simulink model "LUT_kidney_30"  (R2023b)
settings: Solver=FixedStepAuto  StartTime=0  StopTime=10.1  FixedStep=Timegap  RelTol=1e-3
model workspace (MAT data in the model file):
  T1_input = 1.34
(part 3 of 3)

== system LUT_kidney_30/If Action Subsystem6/If Action Subsystem2/If Action Subsystem9/If Action Subsystem11 ==
  In1 : Inport
  Action Port : ActionPort  ActionPortLabel=elseif( u1 >= 1.905)
  LUT 1.91RR : Lookup_n-D  NumberOfTableDimensions=1  BreakpointsForDimension1=[413.2483;519.9897;610.675;704.3665;797.694;890.604;983.1818;1075.506;1167.638;1259.622;1351.49;1443.267;1534.971;1626.615;1718.21;1809.765;1901.286]  Table=[400;500;600;700;800;900;1000;1100;1200;1300;1400;1500;1600;1700;1800;1900;2000]  InternalRulePriority=Speed  RndMeth=Simplest
  Out1 : Outport
  wires:
  In1/1 -> LUT 1.91RR/1
  LUT 1.91RR/1 -> Out1/1

== system LUT_kidney_30/If Action Subsystem6/If Action Subsystem2/If Action Subsystem9/If Action Subsystem2 ==
  In1 : Inport
  Action Port : ActionPort  ActionPortLabel=else
  LUT 1.90RR : Lookup_n-D  NumberOfTableDimensions=1  BreakpointsForDimension1=[413.317;520.0649;610.7574;704.4636;797.8115;890.7462;983.3522;1075.708;1167.873;1259.891;1351.795;1443.609;1535.35;1627.033;1718.667;1810.261;1901.822]  Table=[400;500;600;700;800;900;1000;1100;1200;1300;1400;1500;1600;1700;1800;1900;2000]  InternalRulePriority=Speed  RndMeth=Simplest
  Out1 : Outport
  wires:
  In1/1 -> LUT 1.90RR/1
  LUT 1.90RR/1 -> Out1/1

== system LUT_kidney_30/If Action Subsystem6/If Action Subsystem2/If Action Subsystem9/If Action Subsystem3 ==
  In1 : Inport
  Action Port : ActionPort  ActionPortLabel=elseif( u1 >= 1.925)
  LUT 1.93RR : Lookup_n-D  NumberOfTableDimensions=1  BreakpointsForDimension1=[413.1126;519.8417;610.5139;704.1773;797.4656;890.3275;982.8502;1075.115;1167.182;1259.098;1350.896;1442.6;1534.23;1625.798;1717.317;1808.794;1900.237]  Table=[400;500;600;700;800;900;1000;1100;1200;1300;1400;1500;1600;1700;1800;1900;2000]  InternalRulePriority=Speed  RndMeth=Simplest
  Out1 : Outport
  wires:
  In1/1 -> LUT 1.93RR/1
  LUT 1.93RR/1 -> Out1/1

== system LUT_kidney_30/If Action Subsystem6/If Action Subsystem2/If Action Subsystem9/If Action Subsystem4 ==
  In1 : Inport
  Action Port : ActionPort  ActionPortLabel=elseif( u1 >= 1.935)
  LUT 1.94RR : Lookup_n-D  NumberOfTableDimensions=1  BreakpointsForDimension1=[413.0457;519.7691;610.4352;704.0852;797.3546;890.1931;982.6891;1074.924;1166.96;1258.843;1350.606;1442.275;1533.868;1625.4;1716.881;1808.32;1899.724]  Table=[400;500;600;700;800;900;1000;1100;1200;1300;1400;1500;1600;1700;1800;1900;2000]  InternalRulePriority=Speed  RndMeth=Simplest
  Out1 : Outport
  wires:
  In1/1 -> LUT 1.94RR/1
  LUT 1.94RR/1 -> Out1/1

== system LUT_kidney_30/If Action Subsystem6/If Action Subsystem2/If Action Subsystem9/If Action Subsystem5 ==
  In1 : Inport
  Action Port : ActionPort  ActionPortLabel=elseif( u1 >= 1.955)
  LUT 1.96RR : Lookup_n-D  NumberOfTableDimensions=1  BreakpointsForDimension1=[412.9134;519.6263;610.2812;703.9056;797.1386;889.9319;982.3757;1074.553;1166.527;1258.345;1350.041;1441.64;1533.162;1624.621;1716.028;1807.393;1898.722]  Table=[400;500;600;700;800;900;1000;1100;1200;1300;1400;1500;1600;1700;1800;1900;2000]  InternalRulePriority=Speed  RndMeth=Simplest
  Out1 : Outport
  wires:
  In1/1 -> LUT 1.96RR/1
  LUT 1.96RR/1 -> Out1/1

== system LUT_kidney_30/If Action Subsystem6/If Action Subsystem2/If Action Subsystem9/If Action Subsystem6 ==
  In1 : Inport
  Action Port : ActionPort  ActionPortLabel=elseif( u1 >= 1.945)
  LUT 1.95RR : Lookup_n-D  NumberOfTableDimensions=1  BreakpointsForDimension1=[412.9793;519.6973;610.3576;703.9946;797.2456;890.0613;982.5309;1074.737;1166.742;1258.592;1350.321;1441.955;1533.512;1625.007;1716.451;1807.853;1899.219]  Table=[400;500;600;700;800;900;1000;1100;1200;1300;1400;1500;1600;1700;1800;1900;2000]  InternalRulePriority=Speed  RndMeth=Simplest
  Out1 : Outport
  wires:
  In1/1 -> LUT 1.95RR/1
  LUT 1.95RR/1 -> Out1/1

== system LUT_kidney_30/If Action Subsystem6/If Action Subsystem2/If Action Subsystem9/If Action Subsystem7 ==
  In1 : Inport
  Action Port : ActionPort  ActionPortLabel=elseif( u1 >= 1.965)
  LUT 1.97RR : Lookup_n-D  NumberOfTableDimensions=1  BreakpointsForDimension1=[412.8481;519.5561;610.2059;703.8182;797.0336;889.8049;982.2233;1074.373;1166.317;1258.103;1349.766;1441.331;1532.818;1624.241;1715.612;1806.94;1898.232]  Table=[400;500;600;700;800;900;1000;1100;1200;1300;1400;1500;1600;1700;1800;1900;2000]  InternalRulePriority=Speed  RndMeth=Simplest
  Out1 : Outport
  wires:
  In1/1 -> LUT 1.97RR/1
  LUT 1.97RR/1 -> Out1/1

== system LUT_kidney_30/If Action Subsystem6/If Action Subsystem2/If Action Subsystem9/If Action Subsystem8 ==
  In1 : Inport
  Action Port : ActionPort  ActionPortLabel=elseif( u1 >= 1.975)
  LUT 1.98RR : Lookup_n-D  NumberOfTableDimensions=1  BreakpointsForDimension1=[412.7834;519.4867;610.1317;703.7323;796.9305;889.6803;982.0738;1074.196;1166.11;1257.865;1349.495;1441.026;1532.479;1623.867;1715.202;1806.494;1897.749]  Table=[400;500;600;700;800;900;1000;1100;1200;1300;1400;1500;1600;1700;1800;1900;2000]  InternalRulePriority=Speed  RndMeth=Simplest
  Out1 : Outport
  wires:
  In1/1 -> LUT 1.98RR/1
  LUT 1.98RR/1 -> Out1/1

== system LUT_kidney_30/If Action Subsystem6/If Action Subsystem2/If Action Subsystem9/If Action Subsystem9 ==
  In1 : Inport
  Action Port : ActionPort  ActionPortLabel=elseif(u1 >= 1.985)
  LUT 1.99RR : Lookup_n-D  NumberOfTableDimensions=1  BreakpointsForDimension1=[412.7191;519.4181;610.0586;703.6478;796.8293;889.5581;981.9271;1074.022;1165.907;1257.631;1349.229;1440.727;1532.145;1623.498;1714.798;1806.054;1897.273]  Table=[400;500;600;700;800;900;1000;1100;1200;1300;1400;1500;1600;1700;1800;1900;2000]  InternalRulePriority=Speed  RndMeth=Simplest
  Out1 : Outport
  wires:
  In1/1 -> LUT 1.99RR/1
  LUT 1.99RR/1 -> Out1/1

== system LUT_kidney_30/If Action Subsystem6/If Action Subsystem3/If Action Subsystem5/If Action Subsystem1 ==
  In1 : Inport
  Action Port : ActionPort  ActionPortLabel=elseif( u1 >= 0.615)
  LUT 0.62RR : Lookup_n-D  NumberOfTableDimensions=1  BreakpointsForDimension1=[428.1974;545.7526;646.9497;753.5478;860.9281;968.6199;1076.443;1184.289;1292.077;1399.741;1507.217;1614.398;1721.814;1828.354;1934.705;2040.709;2146.328]  Table=[400;500;600;700;800;900;1000;1100;1200;1300;1400;1500;1600;1700;1800;1900;2000]  InternalRulePriority=Speed  RndMeth=Simplest
  Out1 : Outport
  wires:
  In1/1 -> LUT 0.62RR/1
  LUT 0.62RR/1 -> Out1/1

== system LUT_kidney_30/If Action Subsystem6/If Action Subsystem3/If Action Subsystem5/If Action Subsystem10 ==
  In1 : Inport
  Action Port : ActionPort  ActionPortLabel=elseif( u1 >= 0.605)
  LUT 0.61RR : Lookup_n-D  NumberOfTableDimensions=1  BreakpointsForDimension1=[428.4312;545.8922;647.1097;753.8177;861.3559;969.2312;1077.248;1185.285;1293.251;1401.073;1508.677;1615.901;1723.325;1829.962;1936.285;2042.203;2147.679]  Table=[400;500;600;700;800;900;1000;1100;1200;1300;1400;1500;1600;1700;1800;1900;2000]  InternalRulePriority=Speed  RndMeth=Simplest
  Out1 : Outport
  wires:
  In1/1 -> LUT 0.61RR/1
  LUT 0.61RR/1 -> Out1/1

== system LUT_kidney_30/If Action Subsystem6/If Action Subsystem3/If Action Subsystem5/If Action Subsystem2 ==
  In1 : Inport
  Action Port : ActionPort  ActionPortLabel=else
  LUT 0.6RR : Lookup_n-D  NumberOfTableDimensions=1  BreakpointsForDimension1=[428.6987;546.0043;647.2017;753.9879;861.6572;969.6921;1077.879;1186.082;1294.201;1402.149;1509.845;1616.968;1724.511;1831.145;1937.377;2043.141;2148.399]  Table=[400;500;600;700;800;900;1000;1100;1200;1300;1400;1500;1600;1700;1800;1900;2000]  InternalRulePriority=Speed  RndMeth=Simplest
  Out1 : Outport
  wires:
  In1/1 -> LUT 0.6RR/1
  LUT 0.6RR/1 -> Out1/1

== system LUT_kidney_30/If Action Subsystem6/If Action Subsystem3/If Action Subsystem5/If Action Subsystem3 ==
  In1 : Inport
  Action Port : ActionPort  ActionPortLabel=elseif( u1 >= 0.625)
  LUT 0.63RR : Lookup_n-D  NumberOfTableDimensions=1  BreakpointsForDimension1=[427.9914;545.5872;646.7294;753.1904;860.3904;967.8787;1075.489;1183.124;1290.711;1398.191;1505.511;1612.588;1715.429;1826.388;1932.712;2038.744;2144.441]  Table=[400;500;600;700;800;900;1000;1100;1200;1300;1400;1500;1600;1700;1800;1900;2000]  InternalRulePriority=Speed  RndMeth=Simplest
  Out1 : Outport
  wires:
  In1/1 -> LUT 0.63RR/1
  LUT 0.63RR/1 -> Out1/1

== system LUT_kidney_30/If Action Subsystem6/If Action Subsystem3/If Action Subsystem5/If Action Subsystem4 ==
  In1 : Inport
  Action Port : ActionPort  ActionPortLabel=elseif( u1 >= 0.635)
  LUT 0.64RR : Lookup_n-D  NumberOfTableDimensions=1  BreakpointsForDimension1=[427.808;545.398;646.4556;752.7565;859.7576;967.026;1074.408;1181.814;1289.182;1396.459;1503.597;1610.531;1716.149;1824.126;1930.372;2036.381;2142.102]  Table=[400;500;600;700;800;900;1000;1100;1200;1300;1400;1500;1600;1700;1800;1900;2000]  InternalRulePriority=Speed  RndMeth=Simplest
  Out1 : Outport
  wires:
  In1/1 -> LUT 0.64RR/1
  LUT 0.64RR/1 -> Out1/1

== system LUT_kidney_30/If Action Subsystem6/If Action Subsystem3/If Action Subsystem5/If Action Subsystem5 ==
  In1 : Inport
  Action Port : ActionPort  ActionPortLabel=elseif( u1 >= 0.655)
  LUT 0.66RR : Lookup_n-D  NumberOfTableDimensions=1  BreakpointsForDimension1=[427.4919;544.956;645.7725;751.6992;858.2596;965.0507;1071.94;1178.854;1285.742;1392.564;1499.281;1605.85;1712.098;1818.958;1924.88;2030.721;2136.353]  Table=[400;500;600;700;800;900;1000;1100;1200;1300;1400;1500;1600;1700;1800;1900;2000]  InternalRulePriority=Speed  RndMeth=Simplest
  Out1 : Outport
  wires:
  In1/1 -> LUT 0.66RR/1
  LUT 0.66RR/1 -> Out1/1

== system LUT_kidney_30/If Action Subsystem6/If Action Subsystem3/If Action Subsystem5/If Action Subsystem6 ==
  In1 : Inport
  Action Port : ActionPort  ActionPortLabel=elseif( u1 >= 0.645)
  LUT 0.65RR : Lookup_n-D  NumberOfTableDimensions=1  BreakpointsForDimension1=[427.6427;545.187;646.1347;752.2564;859.0433;966.0784;1073.219;1180.384;1287.518;1394.574;1501.51;1608.272;1714.518;1821.628;1927.744;2033.688;2139.384]  Table=[400;500;600;700;800;900;1000;1100;1200;1300;1400;1500;1600;1700;1800;1900;2000]  InternalRulePriority=Speed  RndMeth=Simplest
  Out1 : Outport
  wires:
  In1/1 -> LUT 0.65RR/1
  LUT 0.65RR/1 -> Out1/1

== system LUT_kidney_30/If Action Subsystem6/If Action Subsystem3/If Action Subsystem5/If Action Subsystem7 ==
  In1 : Inport
  Action Port : ActionPort  ActionPortLabel=elseif( u1 >= 0.665)
  LUT 0.67RR : Lookup_n-D  NumberOfTableDimensions=1  BreakpointsForDimension1=[427.3522;544.7069;645.3744;751.0932;857.4171;963.9562;1070.586;1177.24;1283.874;1390.451;1496.937;1603.295;1709.417;1816.218;1921.825;2027.529;2133.063]  Table=[400;500;600;700;800;900;1000;1100;1200;1300;1400;1500;1600;1700;1800;1900;2000]  InternalRulePriority=Speed  RndMeth=Simplest
  Out1 : Outport
  wires:
  In1/1 -> LUT 0.67RR/1
  LUT 0.67RR/1 -> Out1/1

== system LUT_kidney_30/If Action Subsystem6/If Action Subsystem3/If Action Subsystem5/If Action Subsystem8 ==
  In1 : Inport
  Action Port : ActionPort  ActionPortLabel=elseif(u1 >= 0.675)
  LUT 0.68RR : Lookup_n-D  NumberOfTableDimensions=1  BreakpointsForDimension1=[427.2211;544.4415;644.9453;750.4458;856.5257;962.8065;1069.171;1175.56;1281.933;1388.256;1494.501;1600.635;1706.583;1808.339;1918.622;2024.158;2129.564]  Table=[400;500;600;700;800;900;1000;1100;1200;1300;1400;1500;1600;1700;1800;1900;2000]  InternalRulePriority=Speed  RndMeth=Simplest
  Out1 : Outport
  wires:
  In1/1 -> LUT 0.68RR/1
  LUT 0.68RR/1 -> Out1/1

== system LUT_kidney_30/If Action Subsystem6/If Action Subsystem3/If Action Subsystem5/If Action Subsystem9 ==
  In1 : Inport
  Action Port : ActionPort  ActionPortLabel=if(u1 >= 0.685)
  LUT 0.69RR : Lookup_n-D  NumberOfTableDimensions=1  BreakpointsForDimension1=[427.0963;544.1615;644.4895;749.7638;855.594;961.6121;1067.708;1173.828;1279.934;1385.997;1491.993;1597.893;1703.64;1808.121;1915.309;2020.646;2125.899]  Table=[400;500;600;700;800;900;1000;1100;1200;1300;1400;1500;1600;1700;1800;1900;2000]  InternalRulePriority=Speed  RndMeth=Simplest
  Out1 : Outport
  wires:
  In1/1 -> LUT 0.69RR/1
  LUT 0.69RR/1 -> Out1/1

== system LUT_kidney_30/If Action Subsystem6/If Action Subsystem3/If Action Subsystem6/If Action Subsystem1 ==
  In1 : Inport
  Action Port : ActionPort  ActionPortLabel=elseif( u1 >= 0.515)
  LUT 0.52RR : Lookup_n-D  NumberOfTableDimensions=1  BreakpointsForDimension1=[433.127;545.732;644.4138;749.8879;856.9387;964.7053;1072.719;1180.644;1288.21;1395.177;1501.479;1606.762;1710.998;1814.056;1915.832;2016.24;2115.209]  Table=[400;500;600;700;800;900;1000;1100;1200;1300;1400;1500;1600;1700;1800;1900;2000]  InternalRulePriority=Speed  RndMeth=Simplest
  Out1 : Outport
  wires:
  In1/1 -> LUT 0.52RR/1
  LUT 0.52RR/1 -> Out1/1

== system LUT_kidney_30/If Action Subsystem6/If Action Subsystem3/If Action Subsystem6/If Action Subsystem10 ==
  In1 : Inport
  Action Port : ActionPort  ActionPortLabel=elseif( u1 >= 0.505)
  LUT 0.51RR : Lookup_n-D  NumberOfTableDimensions=1  BreakpointsForDimension1=[434.1573;545.5433;643.469;748.408;855.0555;962.4819;1070.166;1177.73;1284.868;1391.294;1496.956;1601.467;1704.767;1806.718;1907.209;2006.145;2103.45]  Table=[400;500;600;700;800;900;1000;1100;1200;1300;1400;1500;1600;1700;1800;1900;2000]  InternalRulePriority=Speed  RndMeth=Simplest
  Out1 : Outport
  wires:
  In1/1 -> LUT 0.51RR/1
  LUT 0.51RR/1 -> Out1/1

== system LUT_kidney_30/If Action Subsystem6/If Action Subsystem3/If Action Subsystem6/If Action Subsystem2 ==
  In1 : Inport
  Action Port : ActionPort  ActionPortLabel=else
  LUT 0.50RR : Lookup_n-D  NumberOfTableDimensions=1  BreakpointsForDimension1=[435.351;545.3234;642.354;746.6394;852.778;959.7636;1067.016;1174.11;1280.701;1386.344;1491.327;1594.889;1697.058;1797.686;1896.653;1993.856;2089.217]  Table=[400;500;600;700;800;900;1000;1100;1200;1300;1400;1500;1600;1700;1800;1900;2000]  InternalRulePriority=Speed  RndMeth=Simplest
  Out1 : Outport
  wires:
  In1/1 -> LUT 0.50RR/1
  LUT 0.50RR/1 -> Out1/1

== system LUT_kidney_30/If Action Subsystem6/If Action Subsystem3/If Action Subsystem6/If Action Subsystem3 ==
  In1 : Inport
  Action Port : ActionPort  ActionPortLabel=elseif( u1 >= 0.525)
  LUT 0.53RR : Lookup_n-D  NumberOfTableDimensions=1  BreakpointsForDimension1=[432.2397;545.8873;645.2001;751.1029;858.4628;966.4802;1074.733;1182.923;1290.811;1398.189;1502.336;1610.911;1715.912;1819.885;1922.734;2024.382;2124.761]  Table=[400;500;600;700;800;900;1000;1100;1200;1300;1400;1500;1600;1700;1800;1900;2000]  InternalRulePriority=Speed  RndMeth=Simplest
  Out1 : Outport
  wires:
  In1/1 -> LUT 0.53RR/1
  LUT 0.53RR/1 -> Out1/1

== system LUT_kidney_30/If Action Subsystem6/If Action Subsystem3/If Action Subsystem6/If Action Subsystem4 ==
  In1 : Inport
  Action Port : ActionPort  ActionPortLabel=elseif( u1 >= 0.535)
  LUT 0.54RR : Lookup_n-D  NumberOfTableDimensions=1  BreakpointsForDimension1=[431.4769;546.0078;645.8393;752.0761;859.6613;967.8505;1076.263;1184.633;1292.75;1400.431;1506.235;1614.046;1719.658;1824.376;1928.112;2030.794;2132.358]  Table=[400;500;600;700;800;900;1000;1100;1200;1300;1400;1500;1600;1700;1800;1900;2000]  InternalRulePriority=Speed  RndMeth=Simplest
  Out1 : Outport
  wires:
  In1/1 -> LUT 0.54RR/1
  LUT 0.54RR/1 -> Out1/1

== system LUT_kidney_30/If Action Subsystem6/If Action Subsystem3/If Action Subsystem6/If Action Subsystem5 ==
  In1 : Inport
  Action Port : ActionPort  ActionPortLabel=elseif( u1 >= 0.555)
  LUT 0.56RR : Lookup_n-D  NumberOfTableDimensions=1  BreakpointsForDimension1=[430.26;546.1426;646.7222;753.384;861.2069;969.5394;1078.07;1186.589;1294.93;1402.952;1510.471;1617.742;1724.183;1829.965;1934.999;2039.223;2142.587]  Table=[400;500;600;700;800;900;1000;1100;1200;1300;1400;1500;1600;1700;1800;1900;2000]  InternalRulePriority=Speed  RndMeth=Simplest
  Out1 : Outport
  wires:
  In1/1 -> LUT 0.56RR/1
  LUT 0.56RR/1 -> Out1/1

== system LUT_kidney_30/If Action Subsystem6/If Action Subsystem3/If Action Subsystem6/If Action Subsystem6 ==
  In1 : Inport
  Action Port : ActionPort  ActionPortLabel=elseif( u1 >= 0.545)
  LUT 0.55RR : Lookup_n-D  NumberOfTableDimensions=1  BreakpointsForDimension1=[430.822;546.0929;646.343;752.8295;860.5661;968.8574;1077.36;1185.836;1294.1;1401.992;1509.171;1616.285;1722.373;1827.688;1932.145;2035.678;2138.23]  Table=[400;500;600;700;800;900;1000;1100;1200;1300;1400;1500;1600;1700;1800;1900;2000]  InternalRulePriority=Speed  RndMeth=Simplest
  Out1 : Outport
  wires:
  In1/1 -> LUT 0.55RR/1
  LUT 0.55RR/1 -> Out1/1

== system LUT_kidney_30/If Action Subsystem6/If Action Subsystem3/If Action Subsystem6/If Action Subsystem7 ==
  In1 : Inport
  Action Port : ActionPort  ActionPortLabel=elseif( u1 >= 0.565)
  LUT 0.57RR : Lookup_n-D  NumberOfTableDimensions=1  BreakpointsForDimension1=[429.7777;546.1575;646.9876;753.7593;861.6116;969.9322;1078.439;1186.944;1295.3;1403.385;1511.058;1618.528;1725.203;1831.337;1936.821;2041.598;2145.619]  Table=[400;500;600;700;800;900;1000;1100;1200;1300;1400;1500;1600;1700;1800;1900;2000]  InternalRulePriority=Speed  RndMeth=Simplest
  Out1 : Outport
  wires:
  In1/1 -> LUT 0.57RR/1
  LUT 0.57RR/1 -> Out1/1

== system LUT_kidney_30/If Action Subsystem6/If Action Subsystem3/If Action Subsystem6/If Action Subsystem8 ==
  In1 : Inport
  Action Port : ActionPort  ActionPortLabel=elseif(u1 >= 0.575)
  LUT 0.58RR : Lookup_n-D  NumberOfTableDimensions=1  BreakpointsForDimension1=[429.3634;546.1386;647.1496;753.9739;861.806;970.0689;1078.506;1186.949;1295.269;1403.356;1511.097;1614.73;1725.536;1831.922;1937.747;2042.953;2147.499]  Table=[400;500;600;700;800;900;1000;1100;1200;1300;1400;1500;1600;1700;1800;1900;2000]  InternalRulePriority=Speed  RndMeth=Simplest
  Out1 : Outport
  wires:
  In1/1 -> LUT 0.58RR/1
  LUT 0.58RR/1 -> Out1/1

== system LUT_kidney_30/If Action Subsystem6/If Action Subsystem3/If Action Subsystem6/If Action Subsystem9 ==
  In1 : Inport
  Action Port : ActionPort  ActionPortLabel=if(u1 >= 0.585)
  LUT 0.59RR : Lookup_n-D  NumberOfTableDimensions=1  BreakpointsForDimension1=[429.0068;546.087;647.218;754.0448;861.8139;969.9797;1078.308;1186.649;1294.887;1402.926;1510.67;1616.845;1725.276;1831.827;1937.896;2043.427;2148.379]  Table=[400;500;600;700;800;900;1000;1100;1200;1300;1400;1500;1600;1700;1800;1900;2000]  InternalRulePriority=Speed  RndMeth=Simplest
  Out1 : Outport
  wires:
  In1/1 -> LUT 0.59RR/1
  LUT 0.59RR/1 -> Out1/1

== system LUT_kidney_30/If Action Subsystem6/If Action Subsystem3/If Action Subsystem7/If Action Subsystem1 ==
  In1 : Inport
  Action Port : ActionPort  ActionPortLabel=elseif( u1 >= 0.715)
  LUT 0.72RR : Lookup_n-D  NumberOfTableDimensions=1  BreakpointsForDimension1=[426.7421;543.2502;643.001;747.566;852.6291;957.8477;1063.128;1168.429;1273.722;1378.988;1484.209;1589.366;1694.431;1799.282;1905.246;2009.576;2114.25]  Table=[400;500;600;700;800;900;1000;1100;1200;1300;1400;1500;1600;1700;1800;1900;2000]  InternalRulePriority=Speed  RndMeth=Simplest
  Out1 : Outport
  wires:
  In1/1 -> LUT 0.72RR/1
  LUT 0.72RR/1 -> Out1/1

== system LUT_kidney_30/If Action Subsystem6/If Action Subsystem3/If Action Subsystem7/If Action Subsystem10 ==
  In1 : Inport
  Action Port : ActionPort  ActionPortLabel=elseif( u1 >= 0.705)
  LUT 0.71RR : Lookup_n-D  NumberOfTableDimensions=1  BreakpointsForDimension1=[426.8582;543.5643;643.5139;748.3188;853.6393;959.1251;1064.678;1170.252;1275.817;1381.351;1486.833;1592.242;1697.543;1802.536;1908.533;2013.326;2118.212]  Table=[400;500;600;700;800;900;1000;1100;1200;1300;1400;1500;1600;1700;1800;1900;2000]  InternalRulePriority=Speed  RndMeth=Simplest
  Out1 : Outport
  wires:
  In1/1 -> LUT 0.71RR/1
  LUT 0.71RR/1 -> Out1/1

== system LUT_kidney_30/If Action Subsystem6/If Action Subsystem3/If Action Subsystem7/If Action Subsystem2 ==
  In1 : Inport
  Action Port : ActionPort  ActionPortLabel=else
  LUT 0.70RR : Lookup_n-D  NumberOfTableDimensions=1  BreakpointsForDimension1=[426.9758;543.8686;644.0112;749.053;854.6296;960.3823;1066.207;1172.055;1277.891;1383.691;1489.432;1595.089;1700.619;1805.628;1911.928;2017.025;2122.105]  Table=[400;500;600;700;800;900;1000;1100;1200;1300;1400;1500;1600;1700;1800;1900;2000]  InternalRulePriority=Speed  RndMeth=Simplest
  Out1 : Outport
  wires:
  In1/1 -> LUT 0.70RR/1
  LUT 0.70RR/1 -> Out1/1

== system LUT_kidney_30/If Action Subsystem6/If Action Subsystem3/If Action Subsystem7/If Action Subsystem3 ==
  In1 : Inport
  Action Port : ActionPort  ActionPortLabel=elseif( u1 >= 0.725)
  LUT 0.73RR : Lookup_n-D  NumberOfTableDimensions=1  BreakpointsForDimension1=[426.6267;542.9275;642.4753;746.7989;851.6044;956.5563;1061.566;1166.593;1271.616;1376.614;1481.572;1586.475;1691.298;1795.96;1896.303;2005.799;2110.242]  Table=[400;500;600;700;800;900;1000;1100;1200;1300;1400;1500;1600;1700;1800;1900;2000]  InternalRulePriority=Speed  RndMeth=Simplest
  Out1 : Outport
  wires:
  In1/1 -> LUT 0.73RR/1
  LUT 0.73RR/1 -> Out1/1

== system LUT_kidney_30/If Action Subsystem6/If Action Subsystem3/If Action Subsystem7/If Action Subsystem4 ==
  In1 : Inport
  Action Port : ActionPort  ActionPortLabel=elseif( u1 >= 0.735)
  LUT 0.74RR : Lookup_n-D  NumberOfTableDimensions=1  BreakpointsForDimension1=[426.5109;542.5976;641.9396;746.0211;850.5697;955.2565;1059.996;1164.753;1269.505;1374.236;1478.933;1583.58;1688.158;1792.608;1895.708;2002.02;2106.209]  Table=[400;500;600;700;800;900;1000;1100;1200;1300;1400;1500;1600;1700;1800;1900;2000]  InternalRulePriority=Speed  RndMeth=Simplest
  Out1 : Outport
  wires:
  In1/1 -> LUT 0.74RR/1
  LUT 0.74RR/1 -> Out1/1

== system LUT_kidney_30/If Action Subsystem6/If Action Subsystem3/If Action Subsystem7/If Action Subsystem5 ==
  In1 : Inport
  Action Port : ActionPort  ActionPortLabel=elseif( u1 >= 0.755)
  LUT 0.76RR : Lookup_n-D  NumberOfTableDimensions=1  BreakpointsForDimension1=[426.2764;541.9209;640.8473;744.4465;848.4866;952.6498;1056.858;1161.081;1265.3;1369.502;1473.677;1577.814;1681.897;1785.894;1889.567;1994.603;2098.14]  Table=[400;500;600;700;800;900;1000;1100;1200;1300;1400;1500;1600;1700;1800;1900;2000]  InternalRulePriority=Speed  RndMeth=Simplest
  Out1 : Outport
  wires:
  In1/1 -> LUT 0.76RR/1
  LUT 0.76RR/1 -> Out1/1

== system LUT_kidney_30/If Action Subsystem6/If Action Subsystem3/If Action Subsystem7/If Action Subsystem6 ==
  In1 : Inport
  Action Port : ActionPort  ActionPortLabel=elseif( u1 >= 0.745)
  LUT 0.75RR : Lookup_n-D  NumberOfTableDimensions=1  BreakpointsForDimension1=[426.3943;542.2617;641.3963;745.236;849.5293;953.9529;1058.426;1162.914;1267.398;1371.864;1476.298;1580.69;1685.021;1789.248;1892.908;1998.271;2102.17]  Table=[400;500;600;700;800;900;1000;1100;1200;1300;1400;1500;1600;1700;1800;1900;2000]  InternalRulePriority=Speed  RndMeth=Simplest
  Out1 : Outport
  wires:
  In1/1 -> LUT 0.75RR/1
  LUT 0.75RR/1 -> Out1/1

== system LUT_kidney_30/If Action Subsystem6/If Action Subsystem3/If Action Subsystem7/If Action Subsystem7 ==
  In1 : Inport
  Action Port : ActionPort  ActionPortLabel=elseif( u1 >= 0.765)
  LUT 0.77RR : Lookup_n-D  NumberOfTableDimensions=1  BreakpointsForDimension1=[426.1567;541.5762;640.2948;743.6552;847.4448;951.3508;1055.298;1159.259;1263.215;1367.157;1471.074;1574.958;1678.795;1782.558;1886.105;1991.154;2094.134]  Table=[400;500;600;700;800;900;1000;1100;1200;1300;1400;1500;1600;1700;1800;1900;2000]  InternalRulePriority=Speed  RndMeth=Simplest
  Out1 : Outport
  wires:
  In1/1 -> LUT 0.77RR/1
  LUT 0.77RR/1 -> Out1/1

== system LUT_kidney_30/If Action Subsystem6/If Action Subsystem3/If Action Subsystem7/If Action Subsystem8 ==
  In1 : Inport
  Action Port : ActionPort  ActionPortLabel=elseif(u1 >= 0.775)
  LUT 0.78RR : Lookup_n-D  NumberOfTableDimensions=1  BreakpointsForDimension1=[426.035;541.2285;639.7402;742.8643;846.4065;950.0589;1053.749;1157.451;1261.149;1364.833;1468.496;1572.128;1675.719;1779.247;1882.619;1988.504;2090.168]  Table=[400;500;600;700;800;900;1000;1100;1200;1300;1400;1500;1600;1700;1800;1900;2000]  InternalRulePriority=Speed  RndMeth=Simplest
  Out1 : Outport
  wires:
  In1/1 -> LUT 0.78RR/1
  LUT 0.78RR/1 -> Out1/1

== system LUT_kidney_30/If Action Subsystem6/If Action Subsystem3/If Action Subsystem7/If Action Subsystem9 ==
  In1 : Inport
  Action Port : ActionPort  ActionPortLabel=if(u1 >= 0.785)
  LUT 0.79RR : Lookup_n-D  NumberOfTableDimensions=1  BreakpointsForDimension1=[425.9113;540.8787;639.1852;742.0757;845.3741;948.7768;1052.214;1155.661;1259.104;1362.535;1465.946;1569.329;1672.676;1775.969;1879.142;1980.779;2086.259]  Table=[400;500;600;700;800;900;1000;1100;1200;1300;1400;1500;1600;1700;1800;1900;2000]  InternalRulePriority=Speed  RndMeth=Simplest
  Out1 : Outport
  wires:
  In1/1 -> LUT 0.79RR/1
  LUT 0.79RR/1 -> Out1/1

== system LUT_kidney_30/If Action Subsystem6/If Action Subsystem3/If Action Subsystem8/If Action Subsystem1 ==
  In1 : Inport
  Action Port : ActionPort  ActionPortLabel=elseif( u1 >= 0.815)
  LUT 0.82RR : Lookup_n-D  NumberOfTableDimensions=1  BreakpointsForDimension1=[425.5456;539.8244;637.5294;739.7402;842.3309;945.0098;1047.714;1150.423;1253.127;1355.82;1458.498;1561.156;1663.787;1766.382;1868.911;1971.209;2075.321]  Table=[400;500;600;700;800;900;1000;1100;1200;1300;1400;1500;1600;1700;1800;1900;2000]  InternalRulePriority=Speed  RndMeth=Simplest
  Out1 : Outport
  wires:
  In1/1 -> LUT 0.82RR/1
  LUT 0.82RR/1 -> Out1/1

== system LUT_kidney_30/If Action Subsystem6/If Action Subsystem3/If Action Subsystem8/If Action Subsystem10 ==
  In1 : Inport
  Action Port : ActionPort  ActionPortLabel=elseif( u1 >= 0.805)
  LUT 0.81RR : Lookup_n-D  NumberOfTableDimensions=1  BreakpointsForDimension1=[425.6571;540.176;638.0787;740.5124;843.3348;946.2505;1049.195;1152.145;1255.091;1358.026;1460.944;1563.84;1666.707;1769.532;1872.279;1974.668;2078.739]  Table=[400;500;600;700;800;900;1000;1100;1200;1300;1400;1500;1600;1700;1800;1900;2000]  InternalRulePriority=Speed  RndMeth=Simplest
  Out1 : Outport
  wires:
  In1/1 -> LUT 0.81RR/1
  LUT 0.81RR/1 -> Out1/1

== system LUT_kidney_30/If Action Subsystem6/If Action Subsystem3/If Action Subsystem8/If Action Subsystem2 ==
  In1 : Inport
  Action Port : ActionPort  ActionPortLabel=else
  LUT 0.80RR : Lookup_n-D  NumberOfTableDimensions=1  BreakpointsForDimension1=[425.7853;540.5277;638.6309;741.2913;844.3496;947.5067;1050.695;1153.892;1257.084;1360.265;1463.427;1566.566;1669.671;1772.729;1875.692;1978.009;2082.433]  Table=[400;500;600;700;800;900;1000;1100;1200;1300;1400;1500;1600;1700;1800;1900;2000]  InternalRulePriority=Speed  RndMeth=Simplest
  Out1 : Outport
  wires:
  In1/1 -> LUT 0.80RR/1
  LUT 0.80RR/1 -> Out1/1

== system LUT_kidney_30/If Action Subsystem6/If Action Subsystem3/If Action Subsystem8/If Action Subsystem3 ==
  In1 : Inport
  Action Port : ActionPort  ActionPortLabel=elseif( u1 >= 0.825)
  LUT 0.83RR : Lookup_n-D  NumberOfTableDimensions=1  BreakpointsForDimension1=[425.3766;539.4735;636.984;738.976;841.3394;943.7861;1046.255;1148.727;1251.194;1353.65;1456.092;1558.515;1660.914;1763.28;1865.591;1967.739;2072.782]  Table=[400;500;600;700;800;900;1000;1100;1200;1300;1400;1500;1600;1700;1800;1900;2000]  InternalRulePriority=Speed  RndMeth=Simplest
  Out1 : Outport
  wires:
  In1/1 -> LUT 0.83RR/1
  LUT 0.83RR/1 -> Out1/1

== system LUT_kidney_30/If Action Subsystem6/If Action Subsystem3/If Action Subsystem8/If Action Subsystem4 ==
  In1 : Inport
  Action Port : ActionPort  ActionPortLabel=elseif( u1 >= 0.835)
  LUT 0.84RR : Lookup_n-D  NumberOfTableDimensions=1  BreakpointsForDimension1=[425.2593;539.1237;636.4432;738.2206;840.3612;942.5802;1044.819;1147.059;1249.293;1351.516;1453.726;1555.918;1658.089;1760.23;1862.324;1964.296;2064.45]  Table=[400;500;600;700;800;900;1000;1100;1200;1300;1400;1500;1600;1700;1800;1900;2000]  InternalRulePriority=Speed  RndMeth=Simplest
  Out1 : Outport
  wires:
  In1/1 -> LUT 0.84RR/1
  LUT 0.84RR/1 -> Out1/1

== system LUT_kidney_30/If Action Subsystem6/If Action Subsystem3/If Action Subsystem8/If Action Subsystem5 ==
  In1 : Inport
  Action Port : ActionPort  ActionPortLabel=elseif( u1 >= 0.855)
  LUT 0.86RR : Lookup_n-D  NumberOfTableDimensions=1  BreakpointsForDimension1=[424.9841;538.4295;635.3782;736.7393;838.4479;940.2258;1042.018;1143.808;1245.59;1347.362;1449.12;1550.864;1652.589;1754.29;1855.955;1957.544;2058.724]  Table=[400;500;600;700;800;900;1000;1100;1200;1300;1400;1500;1600;1700;1800;1900;2000]  InternalRulePriority=Speed  RndMeth=Simplest
  Out1 : Outport
  wires:
  In1/1 -> LUT 0.86RR/1
  LUT 0.86RR/1 -> Out1/1

== system LUT_kidney_30/If Action Subsystem6/If Action Subsystem3/If Action Subsystem8/If Action Subsystem6 ==
  In1 : Inport
  Action Port : ActionPort  ActionPortLabel=elseif( u1 >= 0.845)
  LUT 0.85RR : Lookup_n-D  NumberOfTableDimensions=1  BreakpointsForDimension1=[425.1226;538.7756;635.9078;737.4748;839.3971;941.3933;1043.406;1145.419;1247.424;1349.42;1451.402;1553.368;1655.313;1757.233;1859.111;1960.895;2061.924]  Table=[400;500;600;700;800;900;1000;1100;1200;1300;1400;1500;1600;1700;1800;1900;2000]  InternalRulePriority=Speed  RndMeth=Simplest
  Out1 : Outport
  wires:
  In1/1 -> LUT 0.85RR/1
  LUT 0.85RR/1 -> Out1/1

== system LUT_kidney_30/If Action Subsystem6/If Action Subsystem3/If Action Subsystem8/If Action Subsystem7 ==
  In1 : Inport
  Action Port : ActionPort  ActionPortLabel=elseif( u1 >= 0.865)
  LUT 0.87RR : Lookup_n-D  NumberOfTableDimensions=1  BreakpointsForDimension1=[424.8438;538.0859;634.8549;736.0145;837.5141;939.0785;1040.654;1142.226;1243.789;1345.342;1446.882;1548.407;1649.915;1751.402;1852.856;1954.248;2055.383]  Table=[400;500;600;700;800;900;1000;1100;1200;1300;1400;1500;1600;1700;1800;1900;2000]  InternalRulePriority=Speed  RndMeth=Simplest
  Out1 : Outport
  wires:
  In1/1 -> LUT 0.87RR/1
  LUT 0.87RR/1 -> Out1/1

== system LUT_kidney_30/If Action Subsystem6/If Action Subsystem3/If Action Subsystem8/If Action Subsystem8 ==
  In1 : Inport
  Action Port : ActionPort  ActionPortLabel=elseif(u1 >= 0.875)
  LUT 0.88RR : Lookup_n-D  NumberOfTableDimensions=1  BreakpointsForDimension1=[424.7021;537.7451;634.3384;735.301;836.596;937.9516;1039.316;1140.674;1242.024;1343.362;1444.687;1545.999;1647.294;1748.569;1849.816;1951.011;2052.028]  Table=[400;500;600;700;800;900;1000;1100;1200;1300;1400;1500;1600;1700;1800;1900;2000]  InternalRulePriority=Speed  RndMeth=Simplest
  Out1 : Outport
  wires:
  In1/1 -> LUT 0.88RR/1
  LUT 0.88RR/1 -> Out1/1

== system LUT_kidney_30/If Action Subsystem6/If Action Subsystem3/If Action Subsystem8/If Action Subsystem9 ==
  In1 : Inport
  Action Port : ActionPort  ActionPortLabel=if(u1 >= 0.885)
  LUT 0.89RR : Lookup_n-D  NumberOfTableDimensions=1  BreakpointsForDimension1=[424.5589;537.4073;633.829;734.5989;835.6941;936.8455;1038.003;1139.153;1240.292;1341.42;1442.536;1543.638;1644.724;1745.792;1846.835;1947.833;2048.701]  Table=[400;500;600;700;800;900;1000;1100;1200;1300;1400;1500;1600;1700;1800;1900;2000]  InternalRulePriority=Speed  RndMeth=Simplest
  Out1 : Outport
  wires:
  In1/1 -> LUT 0.89RR/1
  LUT 0.89RR/1 -> Out1/1

== system LUT_kidney_30/If Action Subsystem6/If Action Subsystem3/If Action Subsystem9/If Action Subsystem1 ==
  In1 : Inport
  Action Port : ActionPort  ActionPortLabel=elseif( u1 >= 0.915)
  LUT 0.92RR : Lookup_n-D  NumberOfTableDimensions=1  BreakpointsForDimension1=[424.1226;536.4147;632.346;732.5645;833.0871;933.6531;1034.217;1134.768;1235.305;1335.83;1436.341;1536.839;1637.324;1737.794;1838.244;1938.664;2039.021]  Table=[400;500;600;700;800;900;1000;1100;1200;1300;1400;1500;1600;1700;1800;1900;2000]  InternalRulePriority=Speed  RndMeth=Simplest
  Out1 : Outport
  wires:
  In1/1 -> LUT 0.92RR/1
  LUT 0.92RR/1 -> Out1/1

== system LUT_kidney_30/If Action Subsystem6/If Action Subsystem3/If Action Subsystem9/If Action Subsystem10 ==
  In1 : Inport
  Action Port : ActionPort  ActionPortLabel=elseif( u1 >= 0.905)
  LUT 0.91RR : Lookup_n-D  NumberOfTableDimensions=1  BreakpointsForDimension1=[424.269;536.7419;632.8326;733.2306;833.9395;934.6962;1035.453;1136.199;1236.933;1337.654;1438.363;1539.058;1639.74;1740.405;1841.049;1941.659;2042.191]  Table=[400;500;600;700;800;900;1000;1100;1200;1300;1400;1500;1600;1700;1800;1900;2000]  InternalRulePriority=Speed  RndMeth=Simplest
  Out1 : Outport
  wires:
  In1/1 -> LUT 0.91RR/1
  LUT 0.91RR/1 -> Out1/1

== system LUT_kidney_30/If Action Subsystem6/If Action Subsystem3/If Action Subsystem9/If Action Subsystem2 ==
  In1 : Inport
  Action Port : ActionPort  ActionPortLabel=else
  LUT 0.90RR : Lookup_n-D  NumberOfTableDimensions=1  BreakpointsForDimension1=[424.4145;537.0728;633.327;733.9087;834.8086;935.7603;1036.715;1137.661;1238.596;1339.518;1440.428;1541.324;1642.206;1743.071;1843.912;1944.716;2045.419]  Table=[400;500;600;700;800;900;1000;1100;1200;1300;1400;1500;1600;1700;1800;1900;2000]  InternalRulePriority=Speed  RndMeth=Simplest
  Out1 : Outport
  wires:
  In1/1 -> LUT 0.90RR/1
  LUT 0.90RR/1 -> Out1/1

== system LUT_kidney_30/If Action Subsystem6/If Action Subsystem3/If Action Subsystem9/If Action Subsystem3 ==
  In1 : Inport
  Action Port : ActionPort  ActionPortLabel=elseif( u1 >= 0.925)
  LUT 0.93RR : Lookup_n-D  NumberOfTableDimensions=1  BreakpointsForDimension1=[423.9754;536.0914;631.8672;731.9107;832.2512;932.6309;1033.005;1133.366;1233.712;1334.043;1434.361;1534.667;1634.959;1735.237;1835.496;1935.73;2035.91]  Table=[400;500;600;700;800;900;1000;1100;1200;1300;1400;1500;1600;1700;1800;1900;2000]  InternalRulePriority=Speed  RndMeth=Simplest
  Out1 : Outport
  wires:
  In1/1 -> LUT 0.93RR/1
  LUT 0.93RR/1 -> Out1/1

== system LUT_kidney_30/If Action Subsystem6/If Action Subsystem3/If Action Subsystem9/If Action Subsystem4 ==
  In1 : Inport
  Action Port : ActionPort  ActionPortLabel=elseif( u1 >= 0.935)
  LUT 0.94RR : Lookup_n-D  NumberOfTableDimensions=1  BreakpointsForDimension1=[423.8275;535.7721;631.3965;731.2692;831.4319;931.6296;1031.819;1131.993;1232.151;1332.294;1432.424;1532.54;1632.644;1732.734;1832.806;1932.855;2032.86]  Table=[400;500;600;700;800;900;1000;1100;1200;1300;1400;1500;1600;1700;1800;1900;2000]  InternalRulePriority=Speed  RndMeth=Simplest
  Out1 : Outport
  wires:
  In1/1 -> LUT 0.94RR/1
  LUT 0.94RR/1 -> Out1/1

== system LUT_kidney_30/If Action Subsystem6/If Action Subsystem3/If Action Subsystem9/If Action Subsystem5 ==
  In1 : Inport
  Action Port : ActionPort  ActionPortLabel=elseif( u1 >= 0.955)
  LUT 0.96RR : Lookup_n-D  NumberOfTableDimensions=1  BreakpointsForDimension1=[423.5306;535.146;630.4794;730.0228;829.8425;929.6888;1029.522;1129.335;1229.13;1328.908;1428.672;1528.423;1628.16;1727.885;1827.595;1927.285;2026.942]  Table=[400;500;600;700;800;900;1000;1100;1200;1300;1400;1500;1600;1700;1800;1900;2000]  InternalRulePriority=Speed  RndMeth=Simplest
  Out1 : Outport
  wires:
  In1/1 -> LUT 0.96RR/1
  LUT 0.96RR/1 -> Out1/1

== system LUT_kidney_30/If Action Subsystem6/If Action Subsystem3/If Action Subsystem9/If Action Subsystem6 ==
  In1 : Inport
  Action Port : ActionPort  ActionPortLabel=elseif( u1 >= 0.945)
  LUT 0.95RR : Lookup_n-D  NumberOfTableDimensions=1  BreakpointsForDimension1=[423.6792;535.4569;630.9339;730.6399;830.629;930.649;1030.658;1130.65;1230.624;1330.583;1430.528;1530.459;1630.378;1730.283;1830.173;1930.041;2029.871]  Table=[400;500;600;700;800;900;1000;1100;1200;1300;1400;1500;1600;1700;1800;1900;2000]  InternalRulePriority=Speed  RndMeth=Simplest
  Out1 : Outport
  wires:
  In1/1 -> LUT 0.95RR/1
  LUT 0.95RR/1 -> Out1/1

== system LUT_kidney_30/If Action Subsystem6/If Action Subsystem3/If Action Subsystem9/If Action Subsystem7 ==
  In1 : Inport
  Action Port : ActionPort  ActionPortLabel=elseif( u1 >= 0.965)
  LUT 0.97RR : Lookup_n-D  NumberOfTableDimensions=1  BreakpointsForDimension1=[423.3817;534.8395;630.033;729.4179;829.0721;928.7488;1028.409;1128.048;1227.667;1327.269;1426.856;1526.43;1625.99;1725.538;1825.072;1924.587;2024.073]  Table=[400;500;600;700;800;900;1000;1100;1200;1300;1400;1500;1600;1700;1800;1900;2000]  InternalRulePriority=Speed  RndMeth=Simplest
  Out1 : Outport
  wires:
  In1/1 -> LUT 0.97RR/1
  LUT 0.97RR/1 -> Out1/1

== system LUT_kidney_30/If Action Subsystem6/If Action Subsystem3/If Action Subsystem9/If Action Subsystem8 ==
  In1 : Inport
  Action Port : ActionPort  ActionPortLabel=elseif(u1 >= 0.975)
  LUT 0.98RR : Lookup_n-D  NumberOfTableDimensions=1  BreakpointsForDimension1=[423.2327;534.5372;629.5947;728.825;828.3178;927.8288;1027.321;1126.789;1226.237;1325.666;1425.08;1524.48;1623.867;1723.241;1822.602;1921.946;2021.264]  Table=[400;500;600;700;800;900;1000;1100;1200;1300;1400;1500;1600;1700;1800;1900;2000]  InternalRulePriority=Speed  RndMeth=Simplest
  Out1 : Outport
  wires:
  In1/1 -> LUT 0.98RR/1
  LUT 0.98RR/1 -> Out1/1

== system LUT_kidney_30/If Action Subsystem6/If Action Subsystem3/If Action Subsystem9/If Action Subsystem9 ==
  In1 : Inport
  Action Port : ActionPort  ActionPortLabel=if(u1 >= 0.985)
  LUT 0.99RR : Lookup_n-D  NumberOfTableDimensions=1  BreakpointsForDimension1=[423.0837;534.2394;629.1645;728.2441;827.5792;926.9283;1026.255;1125.557;1224.837;1324.097;1423.342;1522.572;1621.789;1720.994;1820.185;1919.361;2018.513]  Table=[400;500;600;700;800;900;1000;1100;1200;1300;1400;1500;1600;1700;1800;1900;2000]  InternalRulePriority=Speed  RndMeth=Simplest
  Out1 : Outport
  wires:
  In1/1 -> LUT 0.99RR/1
  LUT 0.99RR/1 -> Out1/1
